simulink model "aero_model"  (R2023b)
settings: Solver=VariableStepAuto  StartTime=0.0  StopTime=10.0  RelTol=1e-3
undefined symbols (not defined in the file or in its folder): a, b
settings Model: Creator=bglen  LastModifiedBy=bglen

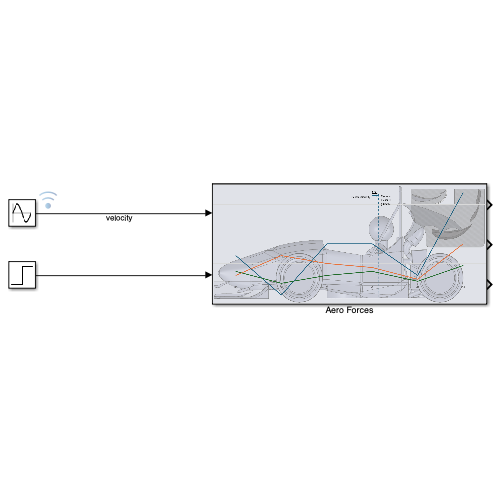
[thumbnail: Simulink's stored preview of the top-level diagram]
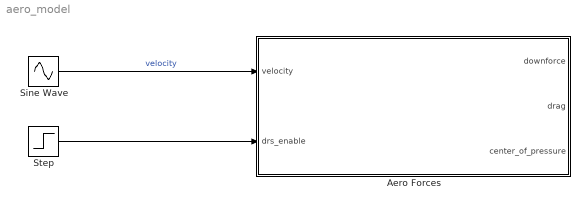
== system aero_model ==
  Aero Forces : Subsystem
      mask Display: image('big_wing.png');
  Sine Wave : Sin  Amplitude=30  Frequency=0.3  SampleTime=0
  Step : Step  Time=3.5  SampleTime=0
  wires:
  Sine Wave/1 -> Aero Forces/1(velocity)  "velocity"
  Step/1 -> Aero Forces/2(drs_enable)

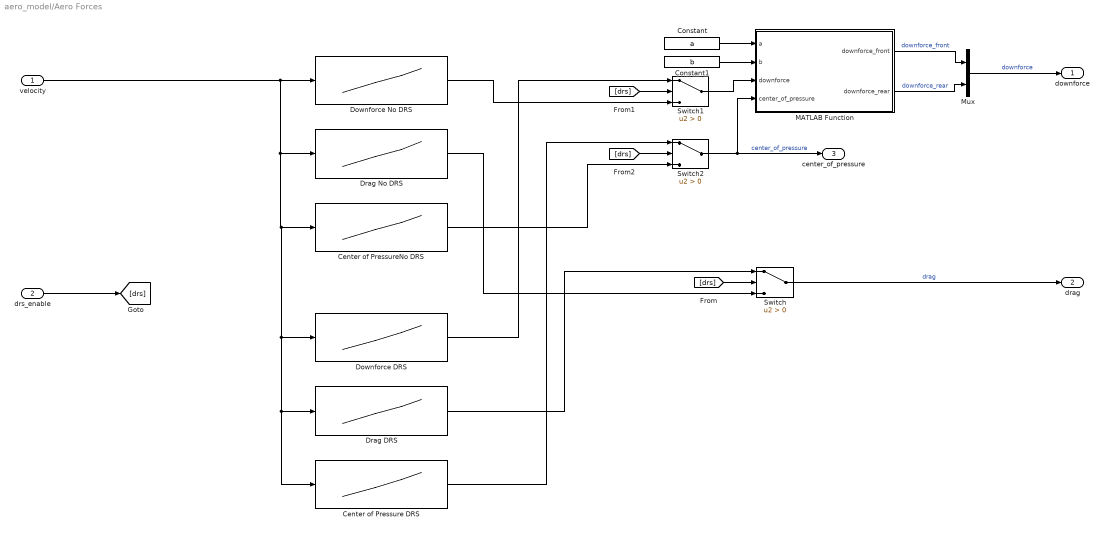
== system aero_model/Aero Forces ==
  velocity : Inport
  drs_enable : Inport  Port=2
  Center of Pressure DRS : Lookup_n-D  NumberOfTableDimensions=1  BreakpointsForDimension1=[2.2352;4.4704;6.7056;8.9408;11.176;13.4112;15.6464;17.8816;20.1168;22.352;24.5872;26.8224;29.0576;31.2928]  Table=[0.176794972966434;0.172602682700208;0.0934978495226155;0.109635046481717;0.0961822849769587;0.0578976665904581;-0.0518352816153028;-0.0850922821311282;-0.112456802684495;-0.110386434440698;-0.121870663573613;-0.172151238551353;-0.185862061581233;-0.199113354149404]  InternalRulePriority=Speed  RndMeth=Simplest
  Center of PressureNo DRS : Lookup_n-D  NumberOfTableDimensions=1  BreakpointsForDimension1=[2.2352;4.4704;6.7056;8.9408;11.176;13.4112;15.6464;17.8816;20.1168;22.352;24.5872;26.8224;29.0576;31.2928]  Table=[-0.135607188802615;-0.137588787703048;-0.195574365979447;-0.215866639322259;-0.22870367751938;-0.278157751621036;-0.366989667896679;-0.310089315236121;-0.333799351635467;-0.289895228213292;-0.377134768583161;-0.440956951229536;-0.50107873320069;-0.516936678234731]  InternalRulePriority=Speed  RndMeth=Simplest
  Constant : Constant  Value=a
  Constant1 : Constant  Value=b
  Downforce DRS : Lookup_n-D  NumberOfTableDimensions=1  BreakpointsForDimension1=[2.2352;4.4704;6.7056;8.9408;11.176;13.4112;15.6464;17.8816;20.1168;22.352;24.5872;26.8224;29.0576;31.2928]  Table=[48.732728255261;71.2374454240421;99.6302490967395;113.50202079035;144.789613578015;217.750213991217;279.051769333153;479.898861584762;694.616494558787;799.328698956136;849.239673042502;860.401352372326;898.870223824537;946.94400741494]  InternalRulePriority=Speed  RndMeth=Simplest
  Downforce No DRS : Lookup_n-D  NumberOfTableDimensions=1  BreakpointsForDimension1=[2.2352;4.4704;6.7056;8.9408;11.176;13.4112;15.6464;17.8816;20.1168;22.352;24.5872;26.8224;29.0576;31.2928]  Table=[67.415259039521;98.5940083581371;133.792591102243;157.005628187984;200.837205930795;313.238609177833;401.822685915433;596.334521302368;902.755723164394;939.369924924251;1159.7623600173;1240.39910819797;1454.89792573704;1551.90214709574]  InternalRulePriority=Speed  RndMeth=Simplest
  Drag DRS : Lookup_n-D  NumberOfTableDimensions=1  BreakpointsForDimension1=[2.2352;4.4704;6.7056;8.9408;11.176;13.4112;15.6464;17.8816;20.1168;22.352;24.5872;26.8224;29.0576;31.2928]  Table=[19.6993853490744;27.57897401486;63.0372609057655;90.6162349206255;118.195208935485;181.232469841251;275.7897401486;334.8087445404;374.274256355665;401.853230370525;571.27086774381;642.195715217825;886.470961759645;984.95547796671]  InternalRulePriority=Speed  RndMeth=Simplest
  Drag No DRS : Lookup_n-D  NumberOfTableDimensions=1  BreakpointsForDimension1=[2.2352;4.4704;6.7056;8.9408;11.176;13.4112;15.6464;17.8816;20.1168;22.352;24.5872;26.8224;29.0576;31.2928]  Table=[22.2411080765;31.1375513071;71.1715458448;102.3090971519;133.446648459;209.0664159191;311.375513071;355.857729224;422.5810534535;453.7186047606;533.786593836;578.268809989;711.715458448;1112.055403825]  InternalRulePriority=Speed  RndMeth=Simplest
  MATLAB Function : MATLAB Function  TreatAsAtomicUnit=on
  Mux : Mux  Inputs=2
  Switch : Switch  Criteria=u2 > Threshold  SaturateOnIntegerOverflow=off  InputSameDT=off
  Switch1 : Switch  Criteria=u2 > Threshold  SaturateOnIntegerOverflow=off  InputSameDT=off
  Switch2 : Switch  Criteria=u2 > Threshold  SaturateOnIntegerOverflow=off  InputSameDT=off
  downforce : Outport
  drag : Outport  Port=2
  center_of_pressure : Outport  Port=3
  wires:
  velocity/1 -> Center of Pressure DRS/1, Drag DRS/1, Downforce DRS/1, Center of PressureNo DRS/1, Drag No DRS/1, Downforce No DRS/1
  Constant1/1 -> MATLAB Function/2(b)
  Constant/1 -> MATLAB Function/1(a)
  MATLAB Function/1(downforce_front) -> Mux/1  "downforce_front"
  MATLAB Function/2(downforce_rear) -> Mux/2  "downforce_rear"
  Mux/1 -> downforce/1  "downforce"
  Switch/1 -> drag/1  "drag"
  Drag No DRS/1 -> Switch/3
  Drag DRS/1 -> Switch/1
  [drs] -> Switch/2
  [drs] -> Switch1/2
  [drs] -> Switch2/2
  Switch1/1 -> MATLAB Function/3(downforce)
  Downforce No DRS/1 -> Switch1/3
  Downforce DRS/1 -> Switch1/1
  Center of PressureNo DRS/1 -> Switch2/3
  Center of Pressure DRS/1 -> Switch2/1
  drs_enable/1 -> [drs]
  Switch2/1 -> MATLAB Function/4(center_of_pressure), center_of_pressure/1  "center_of_pressure"

== matlab function aero_model/Aero Forces/MATLAB Function ==
  data: a input; downforce_front output; b input; downforce input; center_of_pressure input; downforce_rear output
function [downforce_front, downforce_rear] = fcn(a, b, downforce, center_of_pressure)

downforce_front = downforce * (center_of_pressure + b) / (a + b);
downforce_rear = downforce * (a - center_of_pressure) / (a + b);
